simulink model "sampleModel123"  (R2021b)
settings: Solver=VariableStepAuto  StartTime=0.0  StopTime=10.0  RelTol=1e-3
undefined symbols (not defined in the file or in its folder): DiscIntNeverNeededParam
libraries: simulink x4, slpidlib x1
settings Model: Creator=user  LastModifiedBy=user

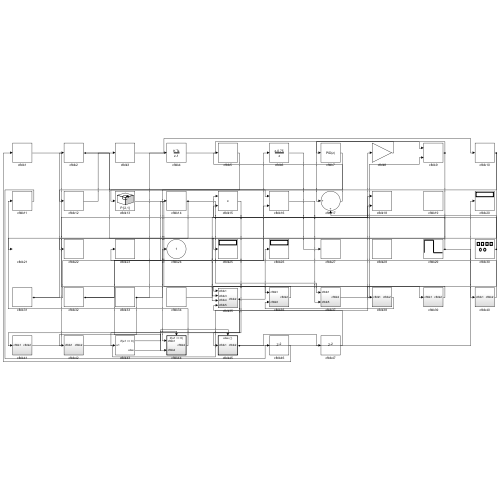
[thumbnail: Simulink's stored preview of the top-level diagram]
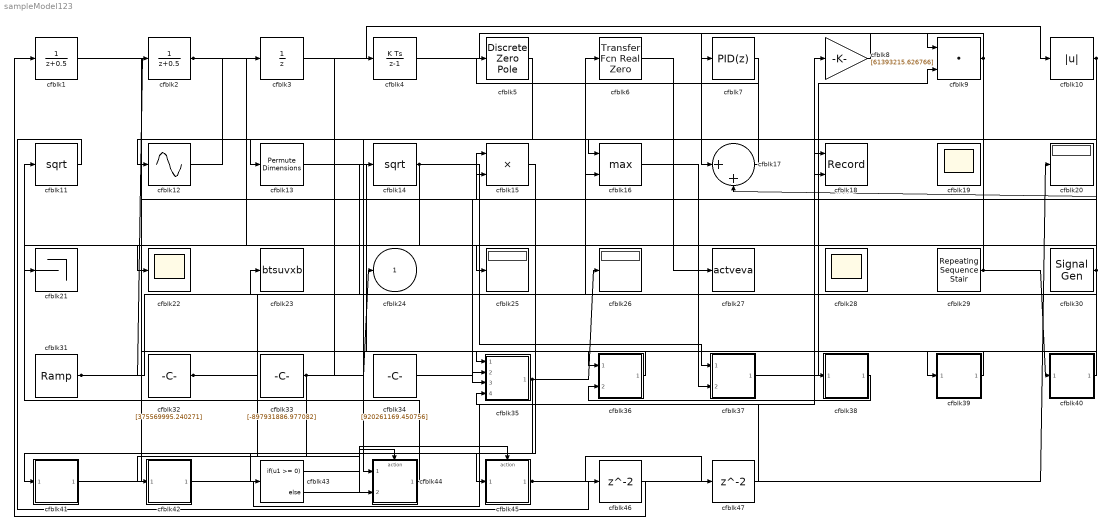
== system sampleModel123 ==
  cfblk1 : DiscreteTransferFcn  SampleTime=1
  cfblk10 : Abs
  cfblk11 : Sqrt  SaturateOnIntegerOverflow=on
  cfblk12 : Sin  TimeSource=Use external signal  SampleTime=0
  cfblk13 : PermuteDimensions
  cfblk14 : Sqrt  SaturateOnIntegerOverflow=on
  cfblk15 : Product
  cfblk16 : MinMax  Function=max  Inputs=2
  cfblk17 : Sum  Inputs=|++
  cfblk18 : Record  FileSettingsInternal="{\"entries\":[{\"content\":{\"excelSettings\":{\"content\":{},\"type\":\"Streamout.ExcelSettings\"}},\"type\":\"Streamout.FileSettingStorage\",\"uuid\":\"7568b358-9aad-4af9-8d11-2ce29c1365cd\"}],\"packageUris\":[\"http://schema.mathworks.com/mf0/streamout_blocks/R2020a\"],\"version\":\"1.0\"}"  Layout=[1 1]  SignalsInternal="{\"entries\":[{\"content\":{\"signals\":[{\"content\":{\"blockPath\":[\"sampleModel123/cfblk18\"],\"channel\":[],\"dimensions\":[1],\"domain\":\"sampleModel123/cfblk18\",\"lineColor\":\"#a2142f\",\"plots\":[1],\"port\":1,\"sid\":[\"\"],\"signalID\":4284,\"signalName\":\"cfblk41\"},\"type\":\"RecordBlkView.Signal\",\"uuid\":\"4af1f1ed-1686-44ad-a446-bba7f3dfda95\"},{\"content\":{\"blockPath\":[\"sampleModel123/cfblk18\"],\"channel\":[],\"dimensions\":[1],\"domain\":\"sampleModel123/cfblk18\",\"lineColor\":\"#139fff\",\"plots\":[1],\"port\":2,\"sid\":[\"\"],\"signalID\":4288,\"signalName\":\"cfblk34\"},\"type\":\"RecordBlkView.Signal\",\"uuid\":\"a0909457-a756-4f15-9201-0aa16580ce4a\"}]},\"type\":\"RecordBlkView.InputSignals\",\"uuid\":\"0848a2e0-f4dc-4c87-9f5e-62bf20c0d9ce\"}],\"packageUris\":[\"http://schema.mathworks.com/mf0/streamout_blocks/R2020a\"],\"version\":\"1.0\"}"  VisualizationBindings="{\"xyplotplugin\":{\"info\":[{\"series\":[{\"bindingParametersList\":[{\"parameter\":\"X-Axis\",\"signalID\":4284,\"signalName\":\"cfblk41\"},{\"parameter\":\"Y-Axis\",\"signalID\":4288,\"signalName\":\"cfblk34\"}],\"seriesID\":28419}],\"subplotID\":1}]}}"  CompatibilityTag=XY
  cfblk19 : Scope
      settings: Floating=on
  cfblk2 : DiscreteTransferFcn  SampleTime=1
  cfblk20 : Display
  cfblk21 : Terminator
  cfblk22 : Scope
  cfblk23 : ToWorkspace  VariableName=btsuvxb  SaveFormat=Timeseries  SampleTime=-1
  cfblk25 : Display
  cfblk26 : Display
  cfblk27 : ToWorkspace  VariableName=actveva  SaveFormat=Timeseries  SampleTime=-1
  cfblk28 : Scope
      settings: Floating=on
  cfblk29 : simulink/Sources/Repeating Sequence Stair  OutValues=[-92777538.356492, -257809128.709867]  tsamp=-1  OutMin=[]  OutMax=[]  OutDataTypeStr=double  OutputDataTypeScalingMode=double  OutDataType=fixdt(0,8)  ConRadixGroup=Best Precision: Vector-wise  OutScaling=2^-12
  cfblk3 : UnitDelay  HasFrameUpgradeWarning=on
  cfblk30 : SignalGenerator  Amplitude=[-148070533.456702]  Units=rad/sec
  cfblk31 : simulink/Sources/Ramp  slope=[-1009.327587]  start=[36.156603]  InitialOutput=[-152936.747057]
  cfblk32 : Constant  Value=[375569995.240271]  SampleTime=1
  cfblk33 : Constant  Value=[-897931886.977082]  SampleTime=1
  cfblk34 : Constant  Value=[920261169.450756]  SampleTime=1
  cfblk35 : Subsystem
  cfblk36 : Subsystem
  cfblk37 : Subsystem
  cfblk38 : Subsystem
  cfblk39 : Subsystem
  cfblk4 : DiscreteIntegrator  ICPrevOutput=DiscIntNeverNeededParam  ICPrevScaledInput=DiscIntNeverNeededParam
  cfblk40 : Subsystem
  cfblk41 : Subsystem
  cfblk42 : Subsystem
  cfblk43 : If  IfExpression=u1 >= 0  SampleTime=1
  cfblk44 : Subsystem  TreatAsAtomicUnit=on
  cfblk45 : Subsystem  TreatAsAtomicUnit=on
  cfblk46 : Delay  SampleTime=1
  cfblk47 : Delay  SampleTime=1
  cfblk5 : DiscreteZeroPole  Poles=[0 0.5]  Gain=1
  cfblk6 : simulink/Discrete/Transfer Fcn Real Zero  ZeroZ=0.75  ICPrevInput=0.0  DoSatur=off
      settings: SourceProductBaseCode=SL
  cfblk7 : slpidlib/PID Controller  Controller=PID  Form=Parallel  TimeDomain=Discrete-time  UseExternalTs=off  SampleTime=1  IntegratorMethod=Forward Euler  FilterMethod=Forward Euler  ControllerParametersSource=internal  P=1  I=1  D=0  UseFilter=on  N=100  TunerSelectOption=Transfer Function Based (PID Tuner App)  InitialConditionSource=internal  InitialConditionForIntegrator=0  InitialConditionForFilter=0  DifferentiatorICPrevScaledInput=0  ExternalReset=none  TrackingMode=off  Kt=1  LimitOutput=off  SatLimitsSource=internal  UpperSaturationLimit=inf  LowerSaturationLimit=-inf  LinearizeAsGain=off  AntiWindupMode=none  Kb=1  POutMin=[]  POutMax=[]  IOutMin=[]  IOutMax=[]  DOutMin=[]  DOutMax=[]  NOutMin=[]  NOutMax=[]  SumOutMin=[]  SumOutMax=[]  SaturationOutMin=[]  SaturationOutMax=[]  PParamMin=[]  PParamMax=[]  IParamMin=[]  IParamMax=[]  DParamMin=[]  DParamMax=[]  NParamMin=[]  NParamMax=[]  KbParamMin=[]  KbParamMax=[]  KtParamMin=[]  KtParamMax=[]  KbOutMin=[]  KbOutMax=[]  KtOutMin=[]  KtOutMax=[]  IntegratorOutMin=[]  IntegratorOutMax=[]  FilterOutMin=[]  FilterOutMax=[]  SumI1OutMin=[]  SumI1OutMax=[]  SumI2OutMin=[]  SumI2OutMax=[]  SumI3OutMin=[]  SumI3OutMax=[]  SumI4OutMin=[]  SumI4OutMax=[]  SumDOutMin=[]  SumDOutMax=[]  DifferentiatorOutMin=[]  DifferentiatorOutMax=[]  FilterDiffOutCoefMin=[]  FilterDiffOutCoefMax=[]  ReciprocalOutMin=[]  ReciprocalOutMax=[]  SumDenOutMin=[]  SumDenOutMax=[]  SumNumOutMin=[]  SumNumOutMax=[]  DivideOutMin=[]  DivideOutMax=[]  UdiffTsProdOutMin=[]  UdiffTsProdOutMax=[]  NTsProdOutMin=[]  NTsProdOutMax=[]  UintegralTsProdOutMin=[]  UintegralTsProdOutMax=[]  UngainTsProdOutMin=[]  UngainTsProdOutMax=[]  IntegratorContinuousStateAttributes=''  IntegratorStateMustResolveToSignalObject=off  IntegratorRTWStateStorageClass=Auto  FilterContinuousStateAttributes=''  FilterStateMustResolveToSignalObject=off  FilterRTWStateStorageClass=Auto  ParallelPVariant=InternalParameters  IdealPVariant=Disabled  IVariant=InternalParameters  DVariant=InternalParameters  IntegratorVariant=Discrete  SatVariant=Disabled  AWVariant=Passthrough  PCopyVariant=Disabled  TRVariant=Disabled  FdbkBlocksVariant=Forward  IdealPFdbkVariant=Disabled  SatFdbkVariant=Disabled  DerivativeFilterVariant=ForwardEulerFilter  NVariant=InternalParameters  NCopyVariant=Disabled  FilterICVariant=InternalICsFilter  IntegratorICVariant=InternalICs  ExternalResetVariant=Disabled  TRSumVariant=Passthrough  SumFdbkVariant=Disabled  SumVariant=Sum_PID  TsampFilterVariant=InternalTs  TsampNgainVariant=Passthrough  TsampIntegralVariant=Passthrough  ExternalSaturationOutDataTypeStr=Inherit: Same as second input
  cfblk8 : Gain  Gain=[61393215.626766]
  cfblk9 : DotProduct  InputSameDT=on  OutDataTypeStr=Inherit: Inherit via internal rule
  cfblk24 : Outport
  wires:
  cfblk44/1(cfblk2) -> cfblk11/1
  cfblk36/1(cfblk2) -> cfblk35/1(cfblk1)
  cfblk45/1(cfblk2) -> cfblk20/1, cfblk47/1
  cfblk42/1(cfblk2) -> cfblk8/1
  cfblk14/1 -> cfblk37/1(cfblk1), cfblk21/1
  cfblk35/1(cfblk2) -> cfblk26/1, cfblk41/1(cfblk1), cfblk43/1
  cfblk6/1 -> cfblk27/1
  cfblk9/1 -> cfblk17/1, cfblk22/1
  cfblk7/1 -> cfblk44/1(cfblk1)
  cfblk40/1(cfblk2) -> cfblk23/1
  cfblk4/1 -> cfblk9/1
  cfblk1/1 -> cfblk36/1(cfblk1)
  cfblk38/1(cfblk2) -> cfblk36/2(cfblk3)
  cfblk8/1 -> cfblk7/1
  cfblk16/1 -> cfblk37/2(cfblk5)
  cfblk15/1 -> cfblk45/1(cfblk1)
  cfblk29/1 -> cfblk40/1(cfblk1), cfblk15/1
  cfblk12/1 -> cfblk3/1
  cfblk30/1 -> cfblk17/2, cfblk35/3(cfblk4), cfblk15/2
  cfblk37/1(cfblk2) -> cfblk9/2
  cfblk13/1 -> cfblk39/1(cfblk1)
  cfblk3/1 -> cfblk10/1
  cfblk41/1(cfblk2) -> cfblk18/1
  cfblk39/1(cfblk2) -> cfblk38/1(cfblk1)
  cfblk31/1 -> cfblk2/1, cfblk6/1
  cfblk34/1 -> cfblk18/2
  cfblk33/1 -> cfblk24/1, cfblk4/1, cfblk42/1(cfblk1)
  cfblk32/1 -> cfblk14/1, cfblk44/2(cfblk4), cfblk16/2
  cfblk2/1 -> cfblk25/1, cfblk16/1
  cfblk17/1 -> cfblk5/1
  cfblk10/1 -> cfblk13/1, cfblk35/2(cfblk3)
  cfblk5/1 -> cfblk12/1
  cfblk43/1 -> cfblk44/Action
  cfblk43/2 -> cfblk45/Action
  cfblk11/1 -> cfblk46/1
  cfblk46/1 -> cfblk1/1
  cfblk47/1 -> cfblk35/4(cfblk5)

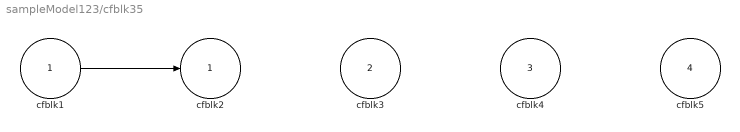
== system sampleModel123/cfblk35 ==
  cfblk1 : Inport
  cfblk3 : Inport  Port=2
  cfblk4 : Inport  Port=3
  cfblk5 : Inport  Port=4
  cfblk2 : Outport
  wires:
  cfblk1/1 -> cfblk2/1

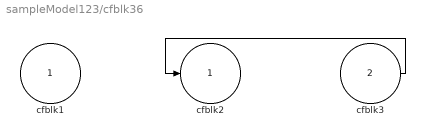
== system sampleModel123/cfblk36 ==
  cfblk1 : Inport
  cfblk3 : Inport  Port=2
  cfblk2 : Outport
  wires:
  cfblk3/1 -> cfblk2/1

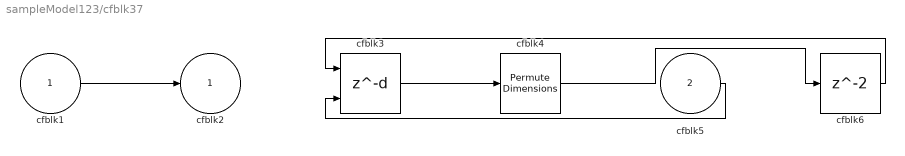
== system sampleModel123/cfblk37 ==
  cfblk1 : Inport
  cfblk5 : Inport  Port=2
  cfblk3 : Delay  DelayLengthSource=Input port  SampleTime=1
      settings: InputPortMap=u0,p1
  cfblk4 : PermuteDimensions
  cfblk6 : Delay  SampleTime=1
  cfblk2 : Outport
  wires:
  cfblk3/1 -> cfblk4/1
  cfblk1/1 -> cfblk2/1
  cfblk5/1 -> cfblk3/2
  cfblk4/1 -> cfblk6/1
  cfblk6/1 -> cfblk3/1

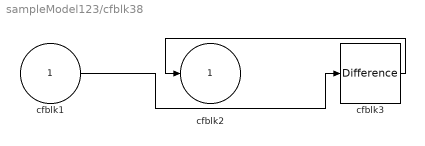
== system sampleModel123/cfblk38 ==
  cfblk1 : Inport
  cfblk3 : simulink/Discrete/Difference  ICPrevInput=0.0  OutMin=[]  OutMax=[]  OutDataTypeStr=Inherit: Inherit via back propagation  OutDataType=fixdt(1, 16)  OutScaling=2^-10  DoSatur=off
  cfblk2 : Outport
  wires:
  cfblk3/1 -> cfblk2/1
  cfblk1/1 -> cfblk3/1

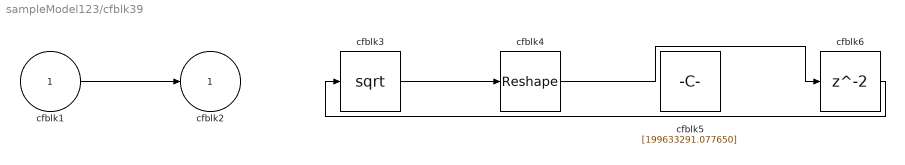
== system sampleModel123/cfblk39 ==
  cfblk1 : Inport
  cfblk3 : Sqrt  SaturateOnIntegerOverflow=on
  cfblk4 : Reshape
  cfblk5 : Constant  Value=[199633291.077650]  SampleTime=1
  cfblk6 : Delay  SampleTime=1
  cfblk2 : Outport
  wires:
  cfblk3/1 -> cfblk4/1
  cfblk1/1 -> cfblk2/1
  cfblk4/1 -> cfblk6/1
  cfblk6/1 -> cfblk3/1

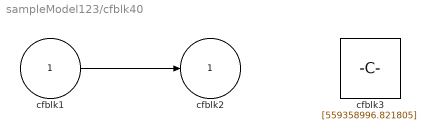
== system sampleModel123/cfblk40 ==
  cfblk1 : Inport
  cfblk3 : Constant  Value=[559358996.821805]  SampleTime=1
  cfblk2 : Outport
  wires:
  cfblk1/1 -> cfblk2/1

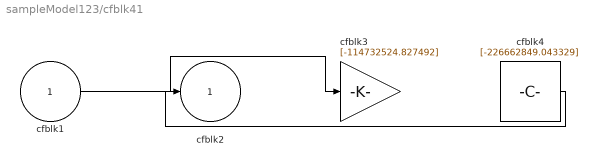
== system sampleModel123/cfblk41 ==
  cfblk1 : Inport
  cfblk3 : Gain  Gain=[-114732524.827492]
  cfblk4 : Constant  Value=[-226662849.043329]  SampleTime=1
  cfblk2 : Outport
  wires:
  cfblk1/1 -> cfblk3/1
  cfblk4/1 -> cfblk2/1

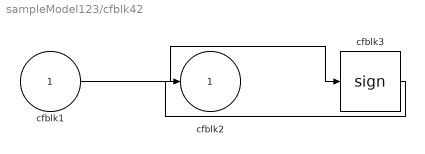
== system sampleModel123/cfblk42 ==
  cfblk1 : Inport
  cfblk3 : Signum
  cfblk2 : Outport
  wires:
  cfblk1/1 -> cfblk3/1
  cfblk3/1 -> cfblk2/1

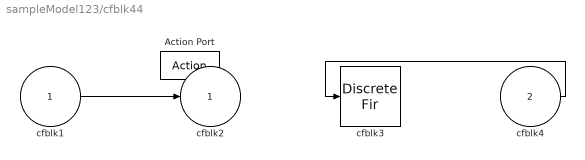
== system sampleModel123/cfblk44 ==
  cfblk1 : Inport
  cfblk4 : Inport  Port=2
  Action Port : ActionPort  ActionPortLabel=if(u1 >= 0)
  cfblk3 : DiscreteFir
  cfblk2 : Outport
  wires:
  cfblk4/1 -> cfblk3/1
  cfblk1/1 -> cfblk2/1

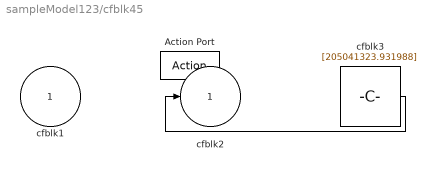
== system sampleModel123/cfblk45 ==
  cfblk1 : Inport
  Action Port : ActionPort  ActionPortLabel=else
  cfblk3 : Constant  Value=[205041323.931988]  SampleTime=1
  cfblk2 : Outport
  wires:
  cfblk3/1 -> cfblk2/1
